simulink model "project_tank_in_series"  (R2019b)
settings: Solver=FixedStepAuto  StartTime=0.0  StopTime=200  RelTol=1e-3
values from neighbouring files (symbols this model uses):
  C = 4.2    [heated_tank_in_series.m]
  rho = 1000    [heated_tank_in_series.m]
  T1 = 4    [heated_tank_in_series.m]
  T2 = 6    [heated_tank_in_series.m]
  UA = 10000    [heated_tank_in_series.m]
  V = 100    [heated_tank_in_series.m]
  w1 = rho*q1    (= 50000)    [heated_tank_in_series.m]
  w2 = rho*q2    (= 50000)    [heated_tank_in_series.m]
undefined symbols (not defined in the file or in its folder): w
settings Model: Creator=oasys  LastModifiedBy=oasys

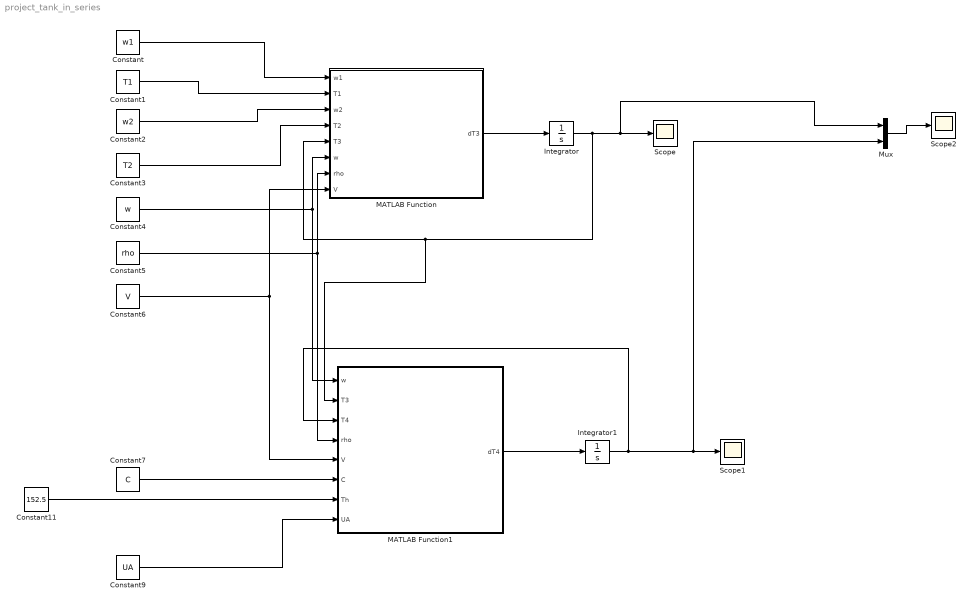
== system project_tank_in_series ==
  Constant : Constant  Value=w1
  Constant1 : Constant  Value=T1
  Constant11 : Constant  Value=152.5
  Constant2 : Constant  Value=w2
  Constant3 : Constant  Value=T2
  Constant4 : Constant  Value=w
  Constant5 : Constant  Value=rho
  Constant6 : Constant  Value=V
  Constant7 : Constant  Value=C
  Constant9 : Constant  Value=UA
  Integrator : Integrator
  Integrator1 : Integrator
  MATLAB Function : MATLAB Function  TreatAsAtomicUnit=on
  MATLAB Function1 : MATLAB Function  TreatAsAtomicUnit=on
  Mux : Mux  Inputs=2
  Scope : Scope
  Scope1 : Scope
  Scope2 : Scope
  wires:
  Constant1/1 -> MATLAB Function/2(T1)
  Constant2/1 -> MATLAB Function/3(w2)
  Constant3/1 -> MATLAB Function/4(T2)
  Constant4/1 -> MATLAB Function1/1(w), MATLAB Function/6(w)
  MATLAB Function/1(dT3) -> Integrator/1
  Integrator/1 -> Mux/1, Scope/1, MATLAB Function/5(T3), MATLAB Function1/2(T3)
  MATLAB Function1/1(dT4) -> Integrator1/1
  Integrator1/1 -> Mux/2, Scope1/1, MATLAB Function1/3(T4)
  Constant5/1 -> MATLAB Function1/4(rho), MATLAB Function/7(rho)
  Constant6/1 -> MATLAB Function/8(V), MATLAB Function1/5(V)
  Constant7/1 -> MATLAB Function1/6(C)
  Constant9/1 -> MATLAB Function1/8(UA)
  Mux/1 -> Scope2/1
  Constant11/1 -> MATLAB Function1/7(Th)
  Constant/1 -> MATLAB Function/1(w1)

== matlab function project_tank_in_series/MATLAB Function1 ==
  data: w input; dT4 output; T3 input; T4 input; rho input; V input; C input; Th input; UA input
function dT4 = T4(w,T3,T4,rho,V,C,Th,UA)
Q = UA*(Th-T4);
dT4 =(w*C*(T3 - T4) + Q)/(rho*V*C);

== matlab function project_tank_in_series/MATLAB Function ==
  data: w1 input; dT3 output; T1 input; w2 input; T2 input; T3 input; w input; rho input; V input
function dT3 = T3(w1,T1,w2,T2,T3,w,rho,V)

dT3 = (T1*w1 + T2*w2 - T3*w)/(rho*V);
